simulink model "Modeling_Fix"  (R2023a)
settings: Solver=VariableStepAuto  StartTime=0.0  StopTime=100  RelTol=1e-3
libraries: slpidlib x1
settings Model: Creator=HP  LastModifiedBy=HP

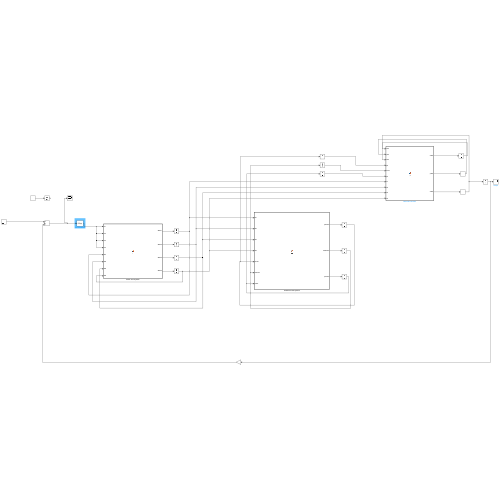
[thumbnail: Simulink's stored preview of the top-level diagram]
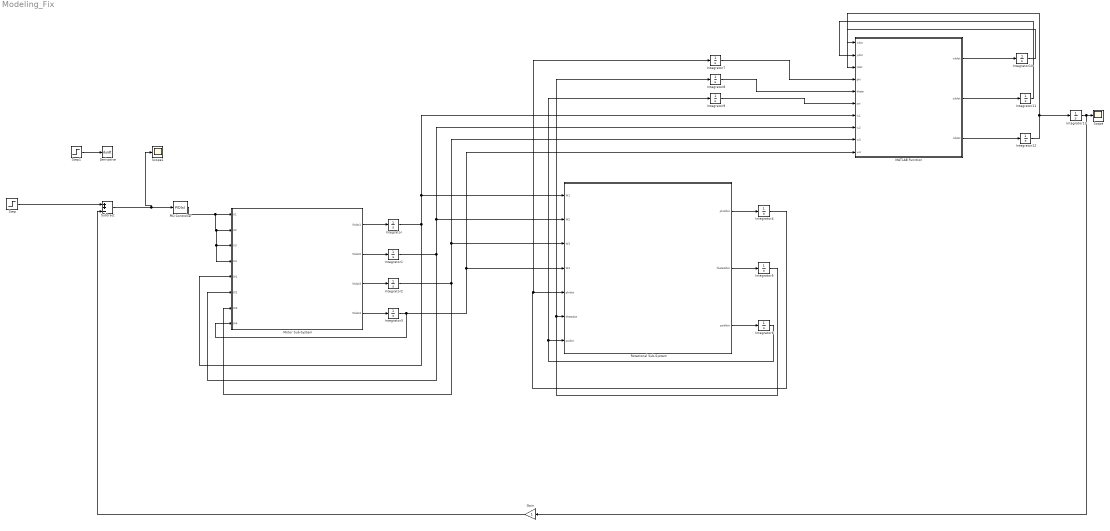
== system Modeling_Fix ==
  Derivative : Derivative
  Gain : Gain
  Integrator{,1..13} (14 alike) : Integrator
  MATLAB Function : MATLAB Function  TreatAsAtomicUnit=on
  Motor Sub-System : MATLAB Function  TreatAsAtomicUnit=on
  PID Controller : slpidlib/PID Controller  Controller=PID  Form=Parallel  TimeDomain=Continuous-time  UseExternalTs=off  SampleTime=-1  IntegratorMethod=Forward Euler  FilterMethod=Forward Euler  ControllerParametersSource=internal  P=0.1  I=1  UseKiTs=off  D=0  N=100  UseFilter=on  TunerSelectOption=Transfer Function Based (PID Tuner App)  InitialConditionSource=internal  InitialConditionForIntegrator=0  InitialConditionForFilter=0  DifferentiatorICPrevScaledInput=0  ExternalReset=none  TrackingMode=off  Kt=1  LimitOutput=off  SatLimitsSource=internal  UpperSaturationLimit=inf  LowerSaturationLimit=-inf  LinearizeAsGain=on  AntiWindupMode=none  Kb=1  LimitIntegrator=off  UpperIntegratorSaturationLimit=inf  LowerIntegratorSaturationLimit=-inf  POutMin=[]  POutMax=[]  IOutMin=[]  IOutMax=[]  DOutMin=[]  DOutMax=[]  NOutMin=[]  NOutMax=[]  SumOutMin=[]  SumOutMax=[]  SaturationOutMin=[]  SaturationOutMax=[]  PParamMin=[]  PParamMax=[]  IParamMin=[]  IParamMax=[]  DParamMin=[]  DParamMax=[]  NParamMin=[]  NParamMax=[]  KbParamMin=[]  KbParamMax=[]  KtParamMin=[]  KtParamMax=[]  KbOutMin=[]  KbOutMax=[]  KtOutMin=[]  KtOutMax=[]  IntegratorOutMin=[]  IntegratorOutMax=[]  FilterOutMin=[]  FilterOutMax=[]  SumI1OutMin=[]  SumI1OutMax=[]  SumI2OutMin=[]  SumI2OutMax=[]  SumI3OutMin=[]  SumI3OutMax=[]  SumI4OutMin=[]  SumI4OutMax=[]  SumDOutMin=[]  SumDOutMax=[]  DifferentiatorOutMin=[]  DifferentiatorOutMax=[]  FilterDiffOutCoefMin=[]  FilterDiffOutCoefMax=[]  ReciprocalOutMin=[]  ReciprocalOutMax=[]  SumDenOutMin=[]  SumDenOutMax=[]  SumNumOutMin=[]  SumNumOutMax=[]  DivideOutMin=[]  DivideOutMax=[]  UdiffTsProdOutMin=[]  UdiffTsProdOutMax=[]  NTsProdOutMin=[]  NTsProdOutMax=[]  UintegralTsProdOutMin=[]  UintegralTsProdOutMax=[]  UngainTsProdOutMin=[]  UngainTsProdOutMax=[]  ClampingZeroOutDataTypeStr=Inherit: Inherit via back propagation  ClampingZeroOutMin=[]  ClampingZeroOutMax=[]  FilterDenConstantOutDataTypeStr=Inherit: Inherit via back propagation  FilterDenConstantOutMin=[]  FilterDenConstantOutMax=[]  PCopyOutDataTypeStr=Inherit: Inherit via back propagation  PCopyOutMin=[]  PCopyOutMax=[]  NCopyOutDataTypeStr=Inherit: Inherit via back propagation  NCopyOutMin=[]  NCopyOutMax=[]  IntegratorContinuousStateAttributes=''  IntegratorStateMustResolveToSignalObject=off  IntegratorRTWStateStorageClass=Auto  FilterContinuousStateAttributes=''  FilterStateMustResolveToSignalObject=off  FilterRTWStateStorageClass=Auto  ParallelPVariant=InternalParameters  IdealPVariant=Disabled  IVariant=InternalParameters  DVariant=InternalParameters  IntegratorVariant=Continuous  SatVariant=Disabled  AWVariant=Passthrough  PCopyVariant=Disabled  TRVariant=Disabled  FdbkBlocksVariant=Forward  IdealPFdbkVariant=Disabled  SatFdbkVariant=Disabled  DerivativeFilterVariant=ContFilter  NVariant=InternalParameters  NCopyVariant=Disabled  FilterICVariant=InternalICsFilter  IntegratorICVariant=InternalICs  ExternalResetVariant=Disabled  TRSumVariant=Passthrough  SumFdbkVariant=Disabled  SumVariant=Sum_PID  TsampFilterVariant=InternalTs  TsampNgainVariant=Passthrough  TsampIntegralVariant=Disabled_SignalSpec  ExternalSaturationOutDataTypeStr=Inherit: Same as second input
  Rotational Sub-System : MATLAB Function  TreatAsAtomicUnit=on
  Scope : Scope
  Scope1 : Scope
  Step : Step  Time=0  SampleTime=0
  Step1 : Step  Time=200  After=99  SampleTime=0
  Subtract : Sum  Inputs=++-
  wires:
  Motor Sub-System/1(Wdot1) -> Integrator/1
  Integrator/1 -> MATLAB Function/7(w1), Rotational Sub-System/1(W1), Motor Sub-System/5(W1)
  Motor Sub-System/2(Wdot2) -> Integrator1/1
  Motor Sub-System/3(Wdot3) -> Integrator2/1
  Motor Sub-System/4(Wdot4) -> Integrator3/1
  Integrator1/1 -> MATLAB Function/8(w2), Rotational Sub-System/2(W2), Motor Sub-System/6(W2)
  Integrator2/1 -> MATLAB Function/9(w3), Rotational Sub-System/3(W3), Motor Sub-System/7(W3)
  Integrator3/1 -> MATLAB Function/10(w4), Rotational Sub-System/4(W4), Motor Sub-System/8(W4)
  Rotational Sub-System/1(phiddot) -> Integrator4/1
  Integrator4/1 -> Integrator7/1, Rotational Sub-System/5(phidot)
  Rotational Sub-System/2(thetaddot) -> Integrator5/1
  Integrator5/1 -> Integrator8/1, Rotational Sub-System/6(thetadot)
  Rotational Sub-System/3(psiddot) -> Integrator6/1
  Integrator6/1 -> Integrator9/1, Rotational Sub-System/7(psidot)
  Integrator7/1 -> MATLAB Function/4(phi)
  Integrator8/1 -> MATLAB Function/5(theta)
  Integrator9/1 -> MATLAB Function/6(psi)
  MATLAB Function/1(xddot) -> Integrator10/1
  Integrator10/1 -> MATLAB Function/1(xdot)
  MATLAB Function/2(yddot) -> Integrator11/1
  Integrator11/1 -> MATLAB Function/2(ydot)
  Integrator12/1 -> MATLAB Function/3(zdot), Integrator13/1
  MATLAB Function/3(zddot) -> Integrator12/1
  Step/1 -> Subtract/1
  Gain/1 -> Subtract/3
  Integrator13/1 -> Gain/1, Scope/1
  Subtract/1 -> PID Controller/1, Scope1/1
  Step1/1 -> Derivative/1
  PID Controller/1 -> Motor Sub-System/4(U4), Motor Sub-System/3(U3), Motor Sub-System/2(U2), Motor Sub-System/1(U1)

== matlab function Modeling_Fix/Rotational Sub-System ==
  data: W1 input; phiddot output; W2 input; W3 input; W4 input; phidot input; thetadot input; psidot input; thetaddot output; psiddot output
function [phiddot, thetaddot, psiddot] = fcn(W1,W2,W3,W4,phidot,thetadot,psidot)
Ixx = 1;
Iyy = 1;
Izz = 1;
l = 1;
alpha = 1; 
beta = 1;
Ca = 1;
CT = 1;
rho = 1;
A = 1;
r =1;

phiddot = ((Iyy - Izz)*(thetadot*psidot) + (W1^2 - W2^2 - W3^2 + W4^2)*0.5*l*sin(alpha)*Ca*rho*A*r^2)/Ixx;
thetaddot = ((Izz - Ixx)*(phidot*psidot) + (W1^2 + W2^2 - W3^2 - W4^2)*0.5*l*sin(beta)*Ca*rho*A*r^2)/Iyy;
psiddot = ((Ixx - Iyy)*(phidot*thetadot) + (-W1^2 + W2^2 - W3^2 + W4^2)*CT*rho*A*r^3)/Izz;

== matlab function Modeling_Fix/Motor Sub-System ==
  data: U1 input; U2 input; U3 input; U4 input; Wdot1 output; Wdot2 output; Wdot3 output; Wdot4 output; W1 input; W2 input; W3 input; W4 input
function [Wdot1,Wdot2,Wdot3,Wdot4] = fcn(U1,U2,U3,U4,W1,W2,W3,W4)
Ke = 1;
Ktm = 1;
Rm =  1;
Jm = 1;
d = 1;
Wo = 1.56524;
n = 1;
r_g = 1;
dm = 1;
A = -(((Ke*Ktm)/(Rm*Jm)) + ((2*d*Wo)/(n*r_g^3*Jm)));
B = Ktm/(Rm*Jm);
C = (dm*Wo^2)/(n*r_g^3*Jm);
Wdot1 = A*W1 + B*U1 + C ;
Wdot2 = A*W2 + B*U2 + C ;
Wdot3 = A*W3 + B*U3 + C ;
Wdot4 = A*W4 + B*U4 + C ;

== matlab function Modeling_Fix/MATLAB Function ==
  data: xdot input; xddot output; ydot input; zdot input; phi input; theta input; psi input; w1 input; w2 input; w3 input; w4 input; yddot output; zddot output
function [xddot,yddot,zddot]= fcn(xdot,ydot,zdot,phi,theta,psi,w1,w2,w3,w4)
Cx = 1;
Cy = 1;
Cz = 1;
Ca = 1;
Ac = 1;
rho = 1;
r = 1;
A = 1;
m = 1;
g = 9.8;

ax = -0.5*Cx*Ac*rho;
ay = -0.5*Cy*Ac*rho;
az = -0.5*Cz*Ac*rho;
wnew = (w1^2+w2^2+w3^2+w4^2);
Ux = (-cos(phi)*sin(theta)*cos(psi)-sin(phi)*sin(psi))*Ca*rho*A*r^2*wnew;
Uy = (-cos(phi)*sin(theta)*cos(psi)+sin(phi)*sin(psi))*Ca*rho*A*r^2*wnew;
Uz = -(cos(phi)*cos(theta))*Ca*rho *A*r^2*wnew;
xddot = (ax*xdot*abs(xdot)+Ux)/m;
yddot = (ay*ydot*abs(ydot)+Uy)/m;
zddot = (az*zdot*abs(zdot)+m*g+Uz)/m;
